simulink model "Tracking"  (R2014b)
settings: Solver=ode45  StartTime=0.0  StopTime=10.0  RelTol=1e-3
undefined symbols (not defined in the file or in its folder): maxNumSigns
libraries: simulink x1
settings Model: Creator=Jackie  LastModifiedBy=Jackie

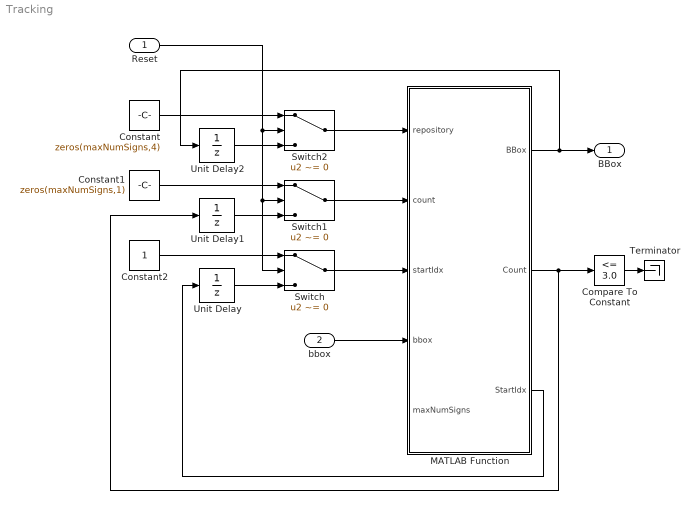
== system Tracking ==
  Reset : Inport
  bbox : Inport  Port=2
  Compare To Constant : simulink/Logic and Bit Operations/Compare To Constant  relop=<=  const=3.0  OutDataTypeStr=boolean
  Constant : Constant  Value=zeros(maxNumSigns,4)
  Constant1 : Constant  Value=zeros(maxNumSigns,1)
  Constant2 : Constant
  MATLAB Function : MATLAB Function  TreatAsAtomicUnit=on
  Switch : Switch  Criteria=u2 ~= 0
  Switch1 : Switch  Criteria=u2 ~= 0
  Switch2 : Switch  Criteria=u2 ~= 0  Threshold=1  OutDataTypeStr=Inherit: Inherit via back propagation  InputSameDT=on
  Terminator : Terminator
  Unit Delay : UnitDelay  SampleTime=-1
  Unit Delay1 : UnitDelay  SampleTime=-1
  Unit Delay2 : UnitDelay  SampleTime=-1
  BBox : Outport
  wires:
  Constant/1 -> Switch2/1
  Unit Delay2/1 -> Switch2/3
  Constant1/1 -> Switch1/1
  Unit Delay1/1 -> Switch1/3
  Constant2/1 -> Switch/1
  Unit Delay/1 -> Switch/3
  Reset/1 -> Switch2/2, Switch1/2, Switch/2
  Switch1/1 -> MATLAB Function/2(count)
  Switch2/1 -> MATLAB Function/1(repository)
  Switch/1 -> MATLAB Function/3(startIdx)
  bbox/1 -> MATLAB Function/4(bbox)
  MATLAB Function/1(BBox) -> BBox/1, Unit Delay2/1
  MATLAB Function/2(Count) -> Unit Delay1/1, Compare To Constant/1
  MATLAB Function/3(StartIdx) -> Unit Delay/1
  Compare To Constant/1 -> Terminator/1

== matlab function Tracking/MATLAB Function ==
  data: repository input; BBox output; count input; startIdx input; bbox input; maxNumSigns input; Count output; StartIdx output
function [BBox, Count, StartIdx] = Match(repository, count, startIdx, bbox, maxNumSigns)
% This function matches the targets found in the current video frame with
% those found in the previous frame. Targets in two video frames match
% when their bounding boxes overlap.
%
% Input:
%    repository: 
%       Bounding boxes of the targets found in the previous
%       frame. Each column has the format of [r, c, h, w] and corresponds 
%       to a target.
%    count: 
%       Number of video frames the target in the previous frame has 
%       been found.
%    startIdx: 
%       Index for the first new target in the current frame.
%    bbox: 
%       Bounding boxes of the targets found in the current frame.
%
% Output:
%    BBox: 
%       Bounding boxes of the targets found in the current frame. They
%       are ordered to have the same indices as their matching ones in the
%       previous frame.
%    Count: 
%       Number of video frames the target in the current frame has 
%       been found.
%    StartIdx: 
%       Index for the first new target in the next frame.

numBBox = single(size(bbox, 1));
BBox = single(zeros(maxNumSigns, 4));
Count = single(zeros(maxNumSigns,1));
impossible = single(10000); % A very large value
thr = single(2);
disMatrix = single(ones(maxNumSigns, numBBox)) * impossible;

% Calculate the distances between the repository and the current targets
for idx = single(1): maxNumSigns
    if repository(idx,3)>0 && repository(idx,4)>0
        for jdx = 1: numBBox
            if bbox(jdx,3)>0 && bbox(jdx,4)>0
                disMatrix(idx, jdx)...
                    = single(abs(2*(repository(idx,1)-bbox(jdx,1))...
                        +repository(idx,3)-bbox(jdx,3))...
                        / (repository(idx,3)+bbox(jdx,3))...
                        + abs(2*(repository(idx,2)-bbox(jdx,2))...
                        +repository(idx,4)-bbox(jdx,4))...
                        / (repository(idx,4)+bbox(jdx,4)));
            end
        end
    end
end

% Find the most similar pair of corners
for n = single(1): numBBox
    minVal = impossible;
    minIdx = single(0);
    minJdx = single(0);
    for idx = 1: single(maxNumSigns)
        for jdx = 1: numBBox
            if disMatrix(idx, jdx) < minVal
                minVal = disMatrix(idx, jdx);
                minIdx = idx;
                minJdx = jdx;
            end
        end
    end
    
    % Move the targets in the current frame so they have the same ordering
    % as their matching ones in the previous frame.
    if minVal < thr
        disMatrix(minIdx, :) = impossible;
        disMatrix(:, minJdx) = impossible;
        BBox(minIdx,:) = bbox(minJdx,:);
        Count(minIdx) = count(minIdx) + 1;
        bbox(minJdx,:) = single(zeros(4, 1));
    else
        break;
    end
end

% Copy the new targets
StartIdx = startIdx;
for jdx = single(1): numBBox
    if bbox(jdx,3)>0
        while BBox(StartIdx,3)
            if StartIdx<maxNumSigns
                StartIdx = StartIdx + single(1);
            else
                StartIdx = single(1);
            end
        end
        BBox(StartIdx, :) = bbox(jdx,:);
        Count(StartIdx) = single(1);
        if StartIdx<maxNumSigns
            StartIdx = StartIdx + single(1);
        else
            StartIdx = single(1);
        end
    end
end
